simulink model "L7M"  (R2020b)
settings: Solver=VariableStepAuto  StartTime=0.0  StopTime=10.0  RelTol=1e-3
undefined symbols (not defined in the file or in its folder): den, num
settings Model: Creator=Julian  LastModifiedBy=Julian

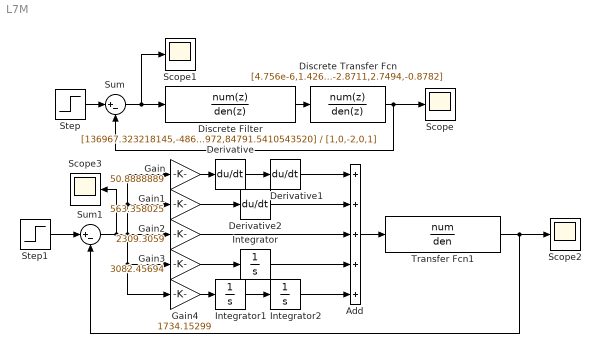
== system L7M ==
  Add : Sum  Inputs=+++++
  Derivative : Derivative
  Derivative1 : Derivative
  Derivative2 : Derivative
  Discrete Transfer Fcn : DiscreteTransferFcn  Numerator=[4.756e-6,1.4268e-5,1.42168e-5,4.75e-6]  Denominator=[1,-2.8711,2.7494,-0.8782]
  Discrete Filter : DiscreteFilter  Numerator=[136967.323218145,-486182.843645550,646802.145617491,-382365.160859972,84791.5410543520]  Denominator=[1,0,-2,0,1]
  Gain : Gain  Gain=50.8888889
  Gain1 : Gain  Gain=563.358025
  Gain2 : Gain  Gain=2309.3059
  Gain3 : Gain  Gain=3082.45694
  Gain4 : Gain  Gain=1734.15299
  Integrator : Integrator
  Integrator1 : Integrator
  Integrator2 : Integrator
  Scope{,1..3} (4 alike) : Scope
  Step : Step  Time=0  SampleTime=0
  Step1 : Step  Time=0  SampleTime=0
  Sum : Sum  Inputs=|+-
  Sum1 : Sum  Inputs=|+-
  Transfer Fcn1 : TransferFcn  Numerator=num  Denominator=den
  wires:
  Sum/1 -> Scope1/1, Discrete Filter/1
  Discrete Filter/1 -> Discrete Transfer Fcn/1
  Discrete Transfer Fcn/1 -> Scope/1, Sum/2
  Step/1 -> Sum/1
  Sum1/1 -> Scope3/1, Gain3/1, Gain4/1, Gain1/1, Gain/1, Gain2/1
  Add/1 -> Transfer Fcn1/1
  Transfer Fcn1/1 -> Scope2/1, Sum1/2
  Step1/1 -> Sum1/1
  Gain/1 -> Derivative/1
  Derivative/1 -> Derivative1/1
  Gain1/1 -> Derivative2/1
  Gain3/1 -> Integrator/1
  Gain4/1 -> Integrator1/1
  Integrator1/1 -> Integrator2/1
  Derivative1/1 -> Add/1
  Derivative2/1 -> Add/2
  Gain2/1 -> Add/3
  Integrator/1 -> Add/4
  Integrator2/1 -> Add/5
